simulink model "Gesamtsystem"  (R2018b)
settings: Solver=FixedStepDiscrete  StartTime=0.0  StopTime=1  RelTol=1e-3  EnableMultiTasking=on
libraries: commutil2 x12, c280xlib x8, c2833xlib x5, powerlib_extras x2, c2000lib x1
(part 1 of 2)
settings Model: ExtModeTrigDuration=8  Creator=User  LastModifiedBy=User
settings DataIOCC: LimitDataPoints=on  SaveFormat=Array  SaveOutput=off  SaveTime=off
settings OptimizationCC: DefaultUnderspecifiedDataType=single  ExpressionDepthLimit=2147483647  LifeSpan=1  MaxStackSize=512
settings DebuggingCC: UnderspecifiedInitializationDetection=Classic  MergeDetectMultiDrivingBlocksExec=none  SolverPrmCheckMsg=warning  StateNameClashWarn=warning  SFUnexpectedBacktrackingDiag=warning  SFNoUnconditionalDefaultTransitionDiag=warning  SFExecutionAtInitializationDiag=none
settings HardwareCC: ProdBitPerChar=16  ProdBitPerInt=16  ProdBitPerPointer=32  ProdBitPerSizeT=32  ProdBitPerPtrDiffT=32  ProdLargestAtomicInteger=Integer  ProdLargestAtomicFloat=None  ProdWordSize=16  ProdLongLongMode=on  ProdHWDeviceType=Texas Instruments->C2000  TargetBitPerChar=16  TargetBitPerInt=16  TargetLargestAtomicInteger=Integer  TargetIntDivRoundTo=Zero  TargetEndianess=LittleEndian  TargetWordSize=16  TargetHWDeviceType=Texas Instruments->C2000  ProdEqTarget=off
settings ModelReferenceCC: PropagateSignalLabelsOutOfModel=off
settings SFSimCC: SimCustomSourceCode="#include \"i2c_reset.c\""  SimCustomHeaderCode="#include \"i2c_reset.h\""  SimUseLocalCustomCode=off  MATLABDynamicMemAlloc=off
settings RTWCC: SystemTargetFile=ert.tlc  HardwareBoard=TI Delfino F2833x  TemplateMakefile=ert_default_tmf  RTWUseLocalCustomCode=off  RTWUseSimCustomCode=on  CustomSourceCode="#include \"i2c_reset.c\""  CustomHeaderCode="#include \"i2c_reset.h\""  Toolchain=Texas Instruments Code Composer Studio (C2000)
settings CodeAppCC: IgnoreCustomStorageClasses=off  CustomSymbolStrType=$N$R$M  StateflowObjectComments=on  InternalIdentifier=Classic
settings ERTTargetCC: CodeReplacementLibrary=TI C28x  MultiwordLength=2048  ParMdlRefBuildCompliant=off  CPPClassGenCompliant=off  ConvertIfToSwitch=off  SuppressUnreachableDefaultCases=off
settings ConfigComp: CovMetricSettings=dw  CovHtmlReporting=on  CovSaveCumulativeToWorkspaceVar=on  CovSaveSingleToWorkspaceVar=on  CovExternalEMLEnable=off  PSAutoStubLUT=on

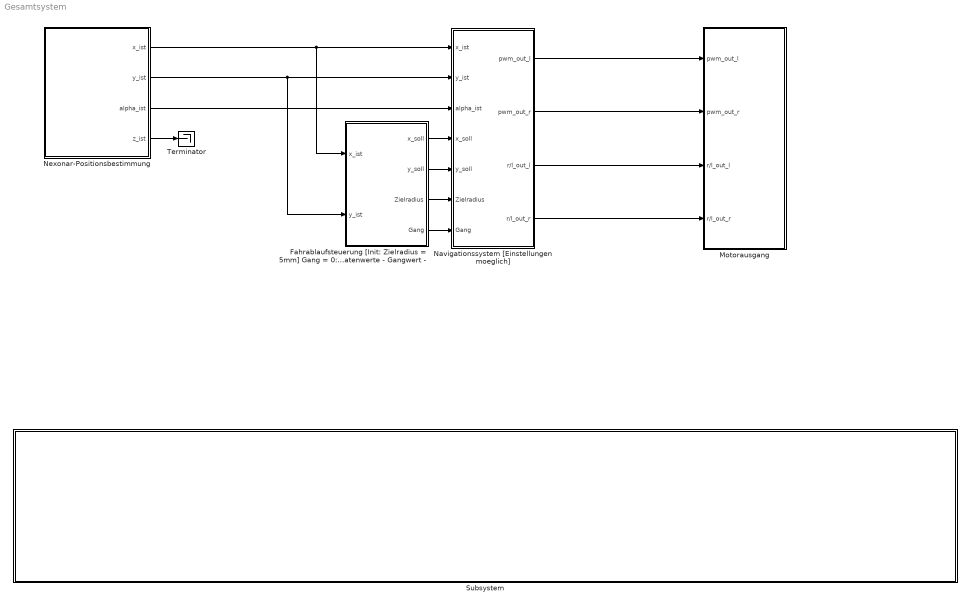
== system Gesamtsystem ==
  "Fahrablaufsteuerung [Init: Zielradius = 5mm] Gang = 0: vorwaerts Gang = 1: rueckwaerts Folgende Werte fuer den Ablauf sind einstellbar: - Zielkoordinatenwerte - Gangwert - " : Stateflow chart  TreatAsAtomicUnit=on
  Motorausgang : Subsystem
  Navigationssystem [Einstellungen moeglich] : Subsystem  TreatAsAtomicUnit=on
  Nexonar-Positionsbestimmung : Subsystem
  Subsystem : Subsystem
  Terminator : Terminator
  wires:
  "Fahrablaufsteuerung [Init: Zielradius = 5mm] Gang = 0: vorwaerts Gang = 1: rueckwaerts Folgende Werte fuer den Ablauf sind einstellbar: - Zielkoordinatenwerte - Gangwert - "/4(Gang) -> Navigationssystem [Einstellungen moeglich]/7(Gang)
  Nexonar-Positionsbestimmung/1(x_ist) -> "Fahrablaufsteuerung [Init: Zielradius = 5mm] Gang = 0: vorwaerts Gang = 1: rueckwaerts Folgende Werte fuer den Ablauf sind einstellbar: - Zielkoordinatenwerte - Gangwert - "/1(x_ist), Navigationssystem [Einstellungen moeglich]/1(x_ist)
  Nexonar-Positionsbestimmung/4(z_ist) -> Terminator/1
  Navigationssystem [Einstellungen moeglich]/4(r/l_out_r) -> Motorausgang/4(r/l_out_r)
  Navigationssystem [Einstellungen moeglich]/1(pwm_out_l) -> Motorausgang/1(pwm_out_l)
  Nexonar-Positionsbestimmung/2(y_ist) -> "Fahrablaufsteuerung [Init: Zielradius = 5mm] Gang = 0: vorwaerts Gang = 1: rueckwaerts Folgende Werte fuer den Ablauf sind einstellbar: - Zielkoordinatenwerte - Gangwert - "/2(y_ist), Navigationssystem [Einstellungen moeglich]/2(y_ist)
  "Fahrablaufsteuerung [Init: Zielradius = 5mm] Gang = 0: vorwaerts Gang = 1: rueckwaerts Folgende Werte fuer den Ablauf sind einstellbar: - Zielkoordinatenwerte - Gangwert - "/3(Zielradius) -> Navigationssystem [Einstellungen moeglich]/6(Zielradius)
  "Fahrablaufsteuerung [Init: Zielradius = 5mm] Gang = 0: vorwaerts Gang = 1: rueckwaerts Folgende Werte fuer den Ablauf sind einstellbar: - Zielkoordinatenwerte - Gangwert - "/1(x_soll) -> Navigationssystem [Einstellungen moeglich]/4(x_soll)
  Navigationssystem [Einstellungen moeglich]/2(pwm_out_r) -> Motorausgang/2(pwm_out_r)
  Nexonar-Positionsbestimmung/3(alpha_ist) -> Navigationssystem [Einstellungen moeglich]/3(alpha_ist)
  "Fahrablaufsteuerung [Init: Zielradius = 5mm] Gang = 0: vorwaerts Gang = 1: rueckwaerts Folgende Werte fuer den Ablauf sind einstellbar: - Zielkoordinatenwerte - Gangwert - "/2(y_soll) -> Navigationssystem [Einstellungen moeglich]/5(y_soll)
  Navigationssystem [Einstellungen moeglich]/3(r/l_out_l) -> Motorausgang/3(r/l_out_l)

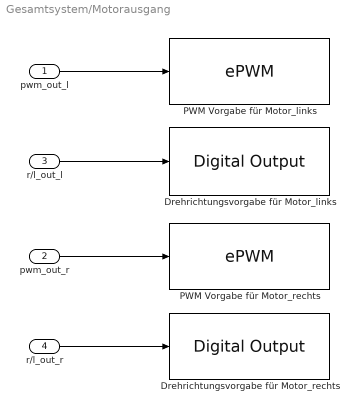
== system Gesamtsystem/Motorausgang ==
  pwm_out_l : Inport
  pwm_out_r : Inport  Port=2
  r/l_out_l : Inport  Port=3
  r/l_out_r : Inport  Port=4
  Drehrichtungsvorgabe für Motor_links : c2833xlib/Digital Output  GPIO_Number=GPIO16~GPIO23  GPIO_Bit0=off  GPIO_BIT0_Toggle=off  GPIO_Bit1=off  GPIO_BIT1_Toggle=off  GPIO_Bit2=off  GPIO_BIT2_Toggle=off  GPIO_Bit3=off  GPIO_BIT3_Toggle=off  GPIO_Bit4=off  GPIO_BIT4_Toggle=off  GPIO_Bit5=on  GPIO_BIT5_Toggle=off  GPIO_Bit6=off  GPIO_BIT6_Toggle=off  GPIO_Bit7=off  GPIO_BIT7_Toggle=off
      settings: SourceProductName=Embedded Coder Support Package for Texas Instruments C2000 Processors  SourceProductBaseCode=TIC2000
  Drehrichtungsvorgabe für Motor_rechts : c2833xlib/Digital Output  GPIO_Number=GPIO16~GPIO23  GPIO_Bit0=off  GPIO_BIT0_Toggle=off  GPIO_Bit1=off  GPIO_BIT1_Toggle=off  GPIO_Bit2=off  GPIO_BIT2_Toggle=off  GPIO_Bit3=off  GPIO_BIT3_Toggle=off  GPIO_Bit4=on  GPIO_BIT4_Toggle=off  GPIO_Bit5=off  GPIO_BIT5_Toggle=off  GPIO_Bit6=off  GPIO_BIT6_Toggle=off  GPIO_Bit7=off  GPIO_BIT7_Toggle=off
      settings: SourceProductName=Embedded Coder Support Package for Texas Instruments C2000 Processors  SourceProductBaseCode=TIC2000
  "PWM Vorgabe für Motor_links " : c280xlib/ePWM  checkMode=off  useModule=ePWM2  periodUnits=Clock cycles  timerSource=Specify via dialog  timerPeriod_clk=64000  timerPeriod_sec=0.0001  tbshadow=Counter equals to zero  countingMode=Up  phaseActiveEnable=Disable  phaseDirection=Count down after sync  phaseActive=0  synchronizationEnable=off  synchronizationOption=Disable  clockPrescale=1  HSclockPrescale=1  ePWMxAStatus=off  CMPAUnits=Clock cycles  CMPASource=Specify via dialog  CMPAValue_per=50  CMPAValue_clk=32000  enCMPAshadow=Counter equals to zero  ePWMxAactionLogic1=Do nothing  ePWMxAactionLogic2=Clear  ePWMxAactionLogic3=Set  ePWMxAactionLogic4=Do nothing  ePWMxAactionLogic5=Do nothing  ePWMxAactionLogic6=Do nothing  ePWMxALoadMode=Load on counter equals to zero (CTR=Zero)  ePWMxACSFenable=off  ePWMxACSFvalue=Forcing disable  ePWMxASFreload=Zero  enHRPWM=off  HRPWM_LoadMode=Counter equals to zero (CTR=ZERO)  HRPWM_CTLMode=Phase control mode  HRPWM_EDGMode=Both edge  enSFO=on  ePWMxBStatus=on  CMPBUnits=Percentages  CMPBSource=Input port  CMPBValue_per=0  CMPBValue_clk=32000  enCMPBshadow=Counter equals to zero  ePWMxBactionLogic1=Do nothing  ePWMxBactionLogic2=Set  ePWMxBactionLogic3=Do nothing  ePWMxBactionLogic4=Do nothing  ePWMxBactionLogic5=Clear  ePWMxBactionLogic6=Do nothing  ePWMxBLoadMode=Load on counter equals to zero (CTR=Zero)  ePWMxBCSFenable=off  ePWMxBCSFvalue=Forcing disable  ePWMxBSFreload=Zero  enableDBePWMxA=off  enableDBePWMxB=off  DBpolarity=Active high (AH)  DBedgeDelay=Positive  DBSource_ePWMxA=ePWMxA  DBSource_ePWMxB=ePWMxA  DBperiodSource=Specify via dialog  REDperiod=0  FEDperiod=0  adcstartModuleA=off  adcrequestEventA=First event  adcstartEventA=Counter equals to zero (CTR=Zero)  adcstartModuleB=off  adcrequestEventB=First event  adcstartEventB=Counter equals to zero (CTR=Zero)  intEn=off  intPrd=First event  intSel=Counter equals to zero (CTR=Zero)  chopperEnable=off  chopperFrequency=1  chopperFirstwidth=1  chopperDuty=12.5%  tripZonesource=Specify via dialog  tzselOSHT1=off  tzselOSHT2=off  tzselOSHT3=off  tzselOSHT4=off  tzselOSHT5=off  tzselOSHT6=off  tzselCBC1=off  tzselCBC2=off  tzselCBC3=off  tzselCBC4=off  tzselCBC5=off  tzselCBC6=off  enTzOstIntr=off  enTzCbcIntr=off  ePWMxAforced=No action  ePWMxBforced=No action  timerPeriod=-1  ePWMxAValue=0  ePWMxBValue=0  tripZoneoption=One-shot trip (OSHT)
      settings: SourceProductName=Embedded Coder Support Package for Texas Instruments C2000 Processors  SourceProductBaseCode=TIC2000
  PWM Vorgabe für Motor_rechts : c280xlib/ePWM  checkMode=off  useModule=ePWM1  periodUnits=Clock cycles  timerSource=Specify via dialog  timerPeriod_clk=64000  timerPeriod_sec=0.0001  tbshadow=Counter equals to zero  countingMode=Up  phaseActiveEnable=Disable  phaseDirection=Count down after sync  phaseActive=0  synchronizationEnable=off  synchronizationOption=Disable  clockPrescale=1  HSclockPrescale=1  ePWMxAStatus=off  CMPAUnits=Clock cycles  CMPASource=Specify via dialog  CMPAValue_per=50  CMPAValue_clk=32000  enCMPAshadow=Counter equals to zero  ePWMxAactionLogic1=Do nothing  ePWMxAactionLogic2=Clear  ePWMxAactionLogic3=Set  ePWMxAactionLogic4=Do nothing  ePWMxAactionLogic5=Do nothing  ePWMxAactionLogic6=Do nothing  ePWMxALoadMode=Load on counter equals to zero (CTR=Zero)  ePWMxACSFenable=off  ePWMxACSFvalue=Forcing disable  ePWMxASFreload=Zero  enHRPWM=off  HRPWM_LoadMode=Counter equals to zero (CTR=ZERO)  HRPWM_CTLMode=Phase control mode  HRPWM_EDGMode=Both edge  enSFO=on  ePWMxBStatus=on  CMPBUnits=Percentages  CMPBSource=Input port  CMPBValue_per=0  CMPBValue_clk=32000  enCMPBshadow=Counter equals to zero  ePWMxBactionLogic1=Do nothing  ePWMxBactionLogic2=Set  ePWMxBactionLogic3=Do nothing  ePWMxBactionLogic4=Do nothing  ePWMxBactionLogic5=Clear  ePWMxBactionLogic6=Do nothing  ePWMxBLoadMode=Load on counter equals to zero (CTR=Zero)  ePWMxBCSFenable=off  ePWMxBCSFvalue=Forcing disable  ePWMxBSFreload=Zero  enableDBePWMxA=off  enableDBePWMxB=off  DBpolarity=Active high (AH)  DBedgeDelay=Positive  DBSource_ePWMxA=ePWMxA  DBSource_ePWMxB=ePWMxA  DBperiodSource=Specify via dialog  REDperiod=0  FEDperiod=0  adcstartModuleA=off  adcrequestEventA=First event  adcstartEventA=Counter equals to zero (CTR=Zero)  adcstartModuleB=off  adcrequestEventB=First event  adcstartEventB=Counter equals to zero (CTR=Zero)  intEn=off  intPrd=First event  intSel=Counter equals to zero (CTR=Zero)  chopperEnable=off  chopperFrequency=1  chopperFirstwidth=1  chopperDuty=12.5%  tripZonesource=Specify via dialog  tzselOSHT1=off  tzselOSHT2=off  tzselOSHT3=off  tzselOSHT4=off  tzselOSHT5=off  tzselOSHT6=off  tzselCBC1=off  tzselCBC2=off  tzselCBC3=off  tzselCBC4=off  tzselCBC5=off  tzselCBC6=off  enTzOstIntr=off  enTzCbcIntr=off  ePWMxAforced=No action  ePWMxBforced=No action  timerPeriod=-1  ePWMxAValue=0  ePWMxBValue=0  tripZoneoption=One-shot trip (OSHT)
      settings: SourceProductName=Embedded Coder Support Package for Texas Instruments C2000 Processors  SourceProductBaseCode=TIC2000
  wires:
  pwm_out_l/1 -> "PWM Vorgabe für Motor_links "/1
  pwm_out_r/1 -> PWM Vorgabe für Motor_rechts/1
  r/l_out_l/1 -> Drehrichtungsvorgabe für Motor_links/1
  r/l_out_r/1 -> Drehrichtungsvorgabe für Motor_rechts/1

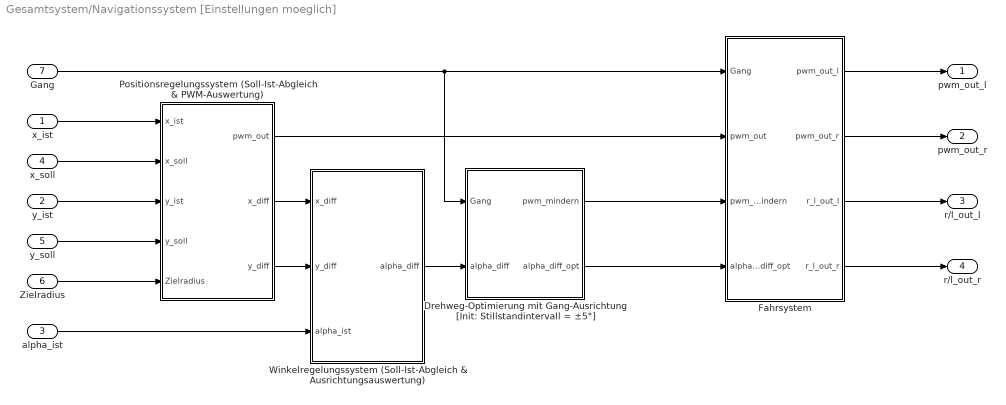
== system Gesamtsystem/Navigationssystem [Einstellungen moeglich] ==
  x_ist : Inport
  y_ist : Inport  Port=2
  alpha_ist : Inport  Port=3
  x_soll : Inport  Port=4
  y_soll : Inport  Port=5
  Zielradius : Inport  Port=6
  Gang : Inport  Port=7
  Drehweg-Optimierung mit Gang-Ausrichtung [Init: Stillstandintervall = ±5°] : Stateflow chart  TreatAsAtomicUnit=on
  Fahrsystem : Stateflow chart  TreatAsAtomicUnit=on
  Positionsregelungssystem (Soll-Ist-Abgleich & PWM-Auswertung) : Subsystem
  Winkelregelungssystem (Soll-Ist-Abgleich & Ausrichtungsauswertung) : Subsystem
  pwm_out_l : Outport
  pwm_out_r : Outport  Port=2
  r/l_out_l : Outport  Port=3
  r/l_out_r : Outport  Port=4
  wires:
  Positionsregelungssystem (Soll-Ist-Abgleich & PWM-Auswertung)/2(x_diff) -> Winkelregelungssystem (Soll-Ist-Abgleich & Ausrichtungsauswertung)/1(x_diff)
  y_soll/1 -> Positionsregelungssystem (Soll-Ist-Abgleich & PWM-Auswertung)/4(y_soll)
  y_ist/1 -> Positionsregelungssystem (Soll-Ist-Abgleich & PWM-Auswertung)/3(y_ist)
  Gang/1 -> Fahrsystem/1(Gang), Drehweg-Optimierung mit Gang-Ausrichtung [Init: Stillstandintervall = ±5°]/1(Gang)
  Positionsregelungssystem (Soll-Ist-Abgleich & PWM-Auswertung)/3(y_diff) -> Winkelregelungssystem (Soll-Ist-Abgleich & Ausrichtungsauswertung)/2(y_diff)
  x_ist/1 -> Positionsregelungssystem (Soll-Ist-Abgleich & PWM-Auswertung)/1(x_ist)
  x_soll/1 -> Positionsregelungssystem (Soll-Ist-Abgleich & PWM-Auswertung)/2(x_soll)
  alpha_ist/1 -> Winkelregelungssystem (Soll-Ist-Abgleich & Ausrichtungsauswertung)/3(alpha_ist)
  Fahrsystem/2(pwm_out_r) -> pwm_out_r/1
  Fahrsystem/4(r_l_out_r) -> r/l_out_r/1
  Fahrsystem/1(pwm_out_l) -> pwm_out_l/1
  Fahrsystem/3(r_l_out_l) -> r/l_out_l/1
  Winkelregelungssystem (Soll-Ist-Abgleich & Ausrichtungsauswertung)/1(alpha_diff) -> Drehweg-Optimierung mit Gang-Ausrichtung [Init: Stillstandintervall = ±5°]/2(alpha_diff)
  Drehweg-Optimierung mit Gang-Ausrichtung [Init: Stillstandintervall = ±5°]/2(alpha_diff_opt) -> Fahrsystem/4(alpha_diff_opt)
  Zielradius/1 -> Positionsregelungssystem (Soll-Ist-Abgleich & PWM-Auswertung)/5(Zielradius)
  Drehweg-Optimierung mit Gang-Ausrichtung [Init: Stillstandintervall = ±5°]/1(pwm_mindern) -> Fahrsystem/3(pwm_mindern)
  Positionsregelungssystem (Soll-Ist-Abgleich & PWM-Auswertung)/1(pwm_out) -> Fahrsystem/2(pwm_out)

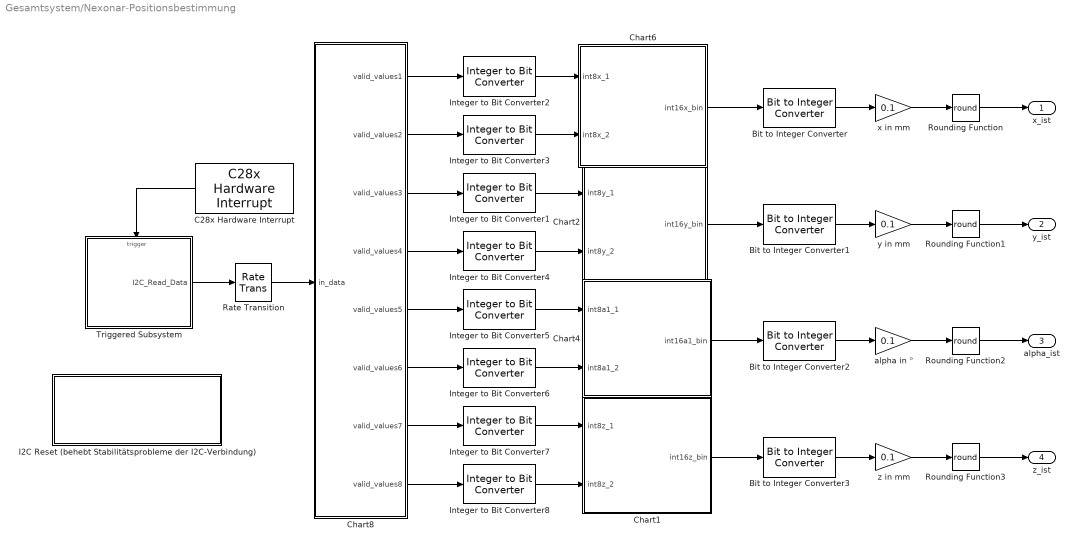
== system Gesamtsystem/Nexonar-Positionsbestimmung ==
  Bit to Integer Converter{,1..3} (4 alike) : commutil2/Bit to Integer Converter  nbits=16  bitOrder=MSB first  signedOutputValues=Signed  outDtype=Inherit via internal rule  outDtypeSigned=Inherit via internal rule
      settings: SourceProductName=Communications Toolbox
  C28x Hardware Interrupt : c2000lib/Scheduling/C28x Hardware Interrupt  irqnumbers=8  pienumbers=2  irqpriorities=30  irqpreempts=0  showinput=off  dspchiptype=C280X
      settings: SourceProductName=Embedded Coder Support Package for Texas Instruments C2000 Processors  SourceProductBaseCode=TIC2000
  Chart1 : Stateflow chart  TreatAsAtomicUnit=on
  Chart2 : Stateflow chart  TreatAsAtomicUnit=on
  Chart4 : Stateflow chart  TreatAsAtomicUnit=on
  Chart6 : Stateflow chart  TreatAsAtomicUnit=on
  Chart8 : Stateflow chart  TreatAsAtomicUnit=on
  I2C Reset (behebt Stabilitätsprobleme der I2C-Verbindung) : Subsystem
  Integer to Bit Converter{1..8} (8 alike) : commutil2/Integer to Bit Converter  nbits=8  signedInputValues=Unsigned  bitOrder=MSB first  outDtype=uint8
      settings: SourceProductName=Communications Toolbox
  Rate Transition : RateTransition  Deterministic=off  OutPortSampleTime=0.01
  Rounding Function{,1..3} (4 alike) : Rounding  Operator=round
  Triggered Subsystem : Subsystem  TreatAsAtomicUnit=on
  alpha in ° : Gain  Gain=0.1  OutDataTypeStr=double
  x in mm : Gain  Gain=0.1  OutDataTypeStr=double
  y in mm : Gain  Gain=0.1  OutDataTypeStr=double
  z in mm : Gain  Gain=0.1  OutDataTypeStr=double
  x_ist : Outport
  y_ist : Outport  Port=2
  alpha_ist : Outport  Port=3
  z_ist : Outport  Port=4
  wires:
  Integer to Bit Converter7/1 -> Chart1/1(int8z_1)
  Integer to Bit Converter8/1 -> Chart1/2(int8z_2)
  Chart8/7(valid_values7) -> Integer to Bit Converter7/1
  Chart8/8(valid_values8) -> Integer to Bit Converter8/1
  Triggered Subsystem/1(I2C_Read_Data) -> Rate Transition/1
  Chart1/1(int16z_bin) -> Bit to Integer Converter3/1
  Chart4/1(int16a1_bin) -> Bit to Integer Converter2/1
  Chart8/6(valid_values6) -> Integer to Bit Converter6/1
  Integer to Bit Converter6/1 -> Chart4/2(int8a1_2)
  Integer to Bit Converter5/1 -> Chart4/1(int8a1_1)
  Integer to Bit Converter4/1 -> Chart2/2(int8y_2)
  Integer to Bit Converter2/1 -> Chart6/1(int8x_1)
  Integer to Bit Converter1/1 -> Chart2/1(int8y_1)
  Chart6/1(int16x_bin) -> Bit to Integer Converter/1
  Integer to Bit Converter3/1 -> Chart6/2(int8x_2)
  Chart8/3(valid_values3) -> Integer to Bit Converter1/1
  Chart8/1(valid_values1) -> Integer to Bit Converter2/1
  Chart2/1(int16y_bin) -> Bit to Integer Converter1/1
  Chart8/4(valid_values4) -> Integer to Bit Converter4/1
  Chart8/2(valid_values2) -> Integer to Bit Converter3/1
  Chart8/5(valid_values5) -> Integer to Bit Converter5/1
  C28x Hardware Interrupt/1 -> Triggered Subsystem/Trigger
  Rate Transition/1 -> Chart8/1(in_data)
  x in mm/1 -> Rounding Function/1
  Bit to Integer Converter/1 -> x in mm/1
  Bit to Integer Converter1/1 -> y in mm/1
  y in mm/1 -> Rounding Function1/1
  Bit to Integer Converter3/1 -> z in mm/1
  z in mm/1 -> Rounding Function3/1
  Bit to Integer Converter2/1 -> alpha in °/1
  alpha in °/1 -> Rounding Function2/1
  Rounding Function/1 -> x_ist/1
  Rounding Function2/1 -> alpha_ist/1
  Rounding Function1/1 -> y_ist/1
  Rounding Function3/1 -> z_ist/1

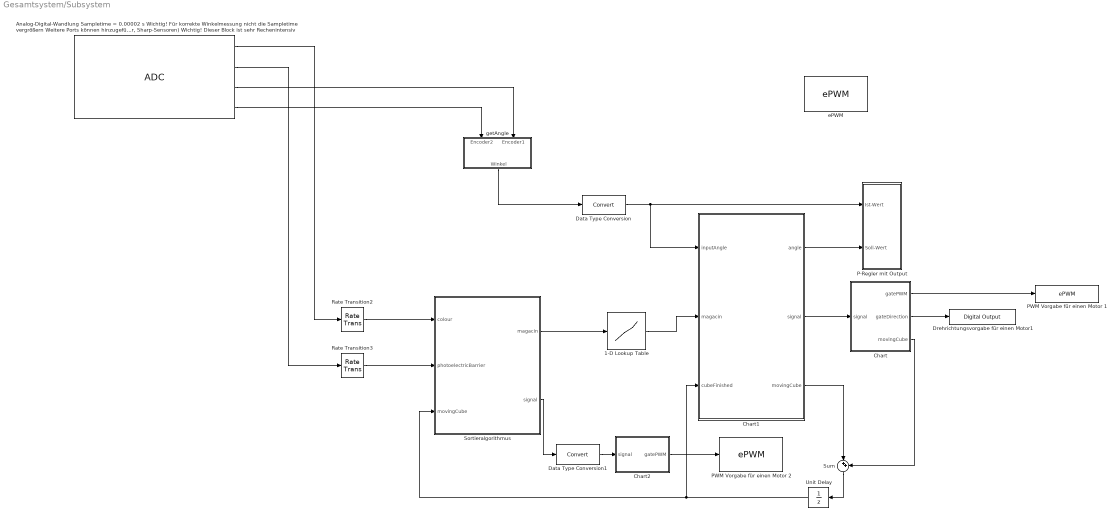
== system Gesamtsystem/Subsystem ==
  1-D Lookup Table : Lookup_n-D  NumberOfTableDimensions=1  BreakpointsForDimension1=[-1,0,1,2,3,4,5,6]  Table=[-1,-440,-295,-170,-40,85,220,430]  InternalRulePriority=Speed  RndMeth=Simplest  InputSameDT=on
  "Analog-Digital-Wandlung Sampletime = 0.00002 s Wichtig! Für korrekte Winkelmessung nicht die Sampletime vergrößern Weitere Ports können hinzugefügt werden (Farbsensor, Sharp-Sensoren) Wichtig! Dieser Block ist sehr Rechenintensiv" : c280xlib/ADC  useModule=A  useMode=Sequential  sourceSOC=Software  sourceSOC1=Software  sourceSOC2=ePWMxB  xint2_ADCSOC=31  Ts=0.00002  dType=double  postInterrupt=off  numConversionsSingle=4  numConversionsDouble=1  conv0=ADCINA0  conv1=ADCINA1  conv2=ADCINA2  conv3=ADCINA3  conv4=ADCINA4  conv5=ADCINA5  conv6=ADCINA6  conv7=ADCINA7  conv8=ADCINB0  conv9=ADCINB1  conv10=ADCINB2  conv11=ADCINB3  conv12=ADCINB4  conv13=ADCINB5  conv14=ADCINB6  conv15=ADCINB7  convAB0=ADCINA0 and ADCINB0  convAB1=ADCINA1 and ADCINB1  convAB2=ADCINA2 and ADCINB2  convAB3=ADCINA3 and ADCINB3  convAB4=ADCINA4 and ADCINB4  convAB5=ADCINA5 and ADCINB5  convAB6=ADCINA6 and ADCINB6  convAB7=ADCINA7 and ADCINB7  convA0=ADCINA5  convA1=ADCINA4  convA2=ADCINA0  convA3=ADCINA1  convA4=ADCINA5  convA5=ADCINA5  convA6=ADCINA6  convA7=ADCINA7  convB0=ADCINB0  convB1=ADCINB1  convB2=ADCINB2  convB3=ADCINB3  convB4=ADCINB4  convB5=ADCINB5  convB6=ADCINB6  convB7=ADCINB7  c28xmultiPort=on  endma=off  chdma=1
      settings: SourceProductName=Embedded Coder Support Package for Texas Instruments C2000 Processors  SourceProductBaseCode=TIC2000
  Chart : Stateflow chart  TreatAsAtomicUnit=on
  Chart1 : Stateflow chart  TreatAsAtomicUnit=on
  Chart2 : Stateflow chart  TreatAsAtomicUnit=on
  Data Type Conversion : DataTypeConversion
  Data Type Conversion1 : DataTypeConversion
  Drehrichtungsvorgabe für einen Motor1 : c2833xlib/Digital Output  GPIO_Number=GPIO16~GPIO23  GPIO_Bit0=on  GPIO_BIT0_Toggle=off  GPIO_Bit1=off  GPIO_BIT1_Toggle=off  GPIO_Bit2=off  GPIO_BIT2_Toggle=off  GPIO_Bit3=off  GPIO_BIT3_Toggle=off  GPIO_Bit4=off  GPIO_BIT4_Toggle=off  GPIO_Bit5=off  GPIO_BIT5_Toggle=off  GPIO_Bit6=off  GPIO_BIT6_Toggle=off  GPIO_Bit7=off  GPIO_BIT7_Toggle=off
      settings: SourceProductName=Embedded Coder Support Package for Texas Instruments C2000 Processors  SourceProductBaseCode=TIC2000
  P-Regler mit Output : Subsystem
  PWM Vorgabe für einen Motor 1 : c280xlib/ePWM  checkMode=off  useModule=ePWM6  periodUnits=Clock cycles  timerSource=Specify via dialog  timerPeriod_clk=64000  timerPeriod_sec=0.0001  tbshadow=Counter equals to zero  countingMode=Up  phaseActiveEnable=Disable  phaseDirection=Count down after sync  phaseActive=0  synchronizationEnable=off  synchronizationOption=Disable  clockPrescale=1  HSclockPrescale=1  ePWMxAStatus=off  CMPAUnits=Clock cycles  CMPASource=Specify via dialog  CMPAValue_per=50  CMPAValue_clk=32000  enCMPAshadow=Counter equals to zero  ePWMxAactionLogic1=Do nothing  ePWMxAactionLogic2=Clear  ePWMxAactionLogic3=Set  ePWMxAactionLogic4=Do nothing  ePWMxAactionLogic5=Do nothing  ePWMxAactionLogic6=Do nothing  ePWMxALoadMode=Load on counter equals to zero (CTR=Zero)  ePWMxACSFenable=off  ePWMxACSFvalue=Forcing disable  ePWMxASFreload=Zero  enHRPWM=off  HRPWM_LoadMode=Counter equals to zero (CTR=ZERO)  HRPWM_CTLMode=Phase control mode  HRPWM_EDGMode=Both edge  enSFO=on  ePWMxBStatus=on  CMPBUnits=Percentages  CMPBSource=Input port  CMPBValue_per=0  CMPBValue_clk=32000  enCMPBshadow=Counter equals to zero  ePWMxBactionLogic1=Do nothing  ePWMxBactionLogic2=Set  ePWMxBactionLogic3=Do nothing  ePWMxBactionLogic4=Do nothing  ePWMxBactionLogic5=Clear  ePWMxBactionLogic6=Do nothing  ePWMxBLoadMode=Load on counter equals to zero (CTR=Zero)  ePWMxBCSFenable=off  ePWMxBCSFvalue=Forcing disable  ePWMxBSFreload=Zero  enableDBePWMxA=off  enableDBePWMxB=off  DBpolarity=Active high (AH)  DBedgeDelay=Positive  DBSource_ePWMxA=ePWMxA  DBSource_ePWMxB=ePWMxA  DBperiodSource=Specify via dialog  REDperiod=0  FEDperiod=0  adcstartModuleA=off  adcrequestEventA=First event  adcstartEventA=Counter equals to zero (CTR=Zero)  adcstartModuleB=off  adcrequestEventB=First event  adcstartEventB=Counter equals to zero (CTR=Zero)  intEn=off  intPrd=First event  intSel=Counter equals to zero (CTR=Zero)  chopperEnable=off  chopperFrequency=1  chopperFirstwidth=1  chopperDuty=12.5%  tripZonesource=Specify via dialog  tzselOSHT1=off  tzselOSHT2=off  tzselOSHT3=off  tzselOSHT4=off  tzselOSHT5=off  tzselOSHT6=off  tzselCBC1=off  tzselCBC2=off  tzselCBC3=off  tzselCBC4=off  tzselCBC5=off  tzselCBC6=off  enTzOstIntr=off  enTzCbcIntr=off  ePWMxAforced=No action  ePWMxBforced=No action  timerPeriod=-1  ePWMxAValue=0  ePWMxBValue=0  tripZoneoption=One-shot trip (OSHT)
      settings: SourceProductName=Embedded Coder Support Package for Texas Instruments C2000 Processors  SourceProductBaseCode=TIC2000
  PWM Vorgabe für einen Motor 2 : c280xlib/ePWM  checkMode=off  useModule=ePWM3  periodUnits=Clock cycles  timerSource=Specify via dialog  timerPeriod_clk=64000  timerPeriod_sec=0.0001  tbshadow=Counter equals to zero  countingMode=Up  phaseActiveEnable=Disable  phaseDirection=Count down after sync  phaseActive=0  synchronizationEnable=off  synchronizationOption=Disable  clockPrescale=1  HSclockPrescale=1  ePWMxAStatus=off  CMPAUnits=Clock cycles  CMPASource=Specify via dialog  CMPAValue_per=50  CMPAValue_clk=32000  enCMPAshadow=Counter equals to zero  ePWMxAactionLogic1=Do nothing  ePWMxAactionLogic2=Clear  ePWMxAactionLogic3=Set  ePWMxAactionLogic4=Do nothing  ePWMxAactionLogic5=Do nothing  ePWMxAactionLogic6=Do nothing  ePWMxALoadMode=Load on counter equals to zero (CTR=Zero)  ePWMxACSFenable=off  ePWMxACSFvalue=Forcing disable  ePWMxASFreload=Zero  enHRPWM=off  HRPWM_LoadMode=Counter equals to zero (CTR=ZERO)  HRPWM_CTLMode=Phase control mode  HRPWM_EDGMode=Both edge  enSFO=on  ePWMxBStatus=on  CMPBUnits=Percentages  CMPBSource=Input port  CMPBValue_per=0  CMPBValue_clk=32000  enCMPBshadow=Counter equals to zero  ePWMxBactionLogic1=Do nothing  ePWMxBactionLogic2=Set  ePWMxBactionLogic3=Do nothing  ePWMxBactionLogic4=Do nothing  ePWMxBactionLogic5=Clear  ePWMxBactionLogic6=Do nothing  ePWMxBLoadMode=Load on counter equals to zero (CTR=Zero)  ePWMxBCSFenable=off  ePWMxBCSFvalue=Forcing disable  ePWMxBSFreload=Zero  enableDBePWMxA=off  enableDBePWMxB=off  DBpolarity=Active high (AH)  DBedgeDelay=Positive  DBSource_ePWMxA=ePWMxA  DBSource_ePWMxB=ePWMxA  DBperiodSource=Specify via dialog  REDperiod=0  FEDperiod=0  adcstartModuleA=off  adcrequestEventA=First event  adcstartEventA=Counter equals to zero (CTR=Zero)  adcstartModuleB=off  adcrequestEventB=First event  adcstartEventB=Counter equals to zero (CTR=Zero)  intEn=off  intPrd=First event  intSel=Counter equals to zero (CTR=Zero)  chopperEnable=off  chopperFrequency=1  chopperFirstwidth=1  chopperDuty=12.5%  tripZonesource=Specify via dialog  tzselOSHT1=off  tzselOSHT2=off  tzselOSHT3=off  tzselOSHT4=off  tzselOSHT5=off  tzselOSHT6=off  tzselCBC1=off  tzselCBC2=off  tzselCBC3=off  tzselCBC4=off  tzselCBC5=off  tzselCBC6=off  enTzOstIntr=off  enTzCbcIntr=off  ePWMxAforced=No action  ePWMxBforced=No action  timerPeriod=-1  ePWMxAValue=0  ePWMxBValue=0  tripZoneoption=One-shot trip (OSHT)
      settings: SourceProductName=Embedded Coder Support Package for Texas Instruments C2000 Processors  SourceProductBaseCode=TIC2000
  Rate Transition2 : RateTransition  OutPortSampleTime=0.01
  Rate Transition3 : RateTransition  OutPortSampleTime=0.01
  Sortieralgorithmus : Stateflow chart  TreatAsAtomicUnit=on
  Sum : Sum  Inputs=|++
  Unit Delay : UnitDelay  SampleTime=-1
  ePWM : c280xlib/ePWM  checkMode=off  useModule=ePWM5  periodUnits=Clock cycles  timerSource=Specify via dialog  timerPeriod_clk=64000  timerPeriod_sec=0.0001  tbshadow=Counter equals to zero  countingMode=Up  phaseActiveEnable=Disable  phaseDirection=Count down after sync  phaseActive=0  synchronizationEnable=off  synchronizationOption=Disable  clockPrescale=1  HSclockPrescale=1  ePWMxAStatus=off  CMPAUnits=Percentages  CMPASource=Specify via dialog  CMPAValue_per=30  CMPAValue_clk=32000  enCMPAshadow=Counter equals to zero  ePWMxAactionLogic1=Do nothing  ePWMxAactionLogic2=Clear  ePWMxAactionLogic3=Set  ePWMxAactionLogic4=Do nothing  ePWMxAactionLogic5=Do nothing  ePWMxAactionLogic6=Do nothing  ePWMxALoadMode=Load on counter equals to zero (CTR=Zero)  ePWMxACSFenable=off  ePWMxACSFvalue=Forcing disable  ePWMxASFreload=Zero  enHRPWM=off  HRPWM_LoadMode=Counter equals to zero (CTR=ZERO)  HRPWM_CTLMode=Phase control mode  HRPWM_EDGMode=Both edge  enSFO=on  ePWMxBStatus=on  CMPBUnits=Percentages  CMPBSource=Specify via dialog  CMPBValue_per=80  CMPBValue_clk=32000  enCMPBshadow=Counter equals to zero  ePWMxBactionLogic1=Do nothing  ePWMxBactionLogic2=Set  ePWMxBactionLogic3=Do nothing  ePWMxBactionLogic4=Do nothing  ePWMxBactionLogic5=Clear  ePWMxBactionLogic6=Do nothing  ePWMxBLoadMode=Load on counter equals to zero (CTR=Zero)  ePWMxBCSFenable=off  ePWMxBCSFvalue=Forcing disable  ePWMxBSFreload=Zero  enableDBePWMxA=off  enableDBePWMxB=off  DBpolarity=Active high (AH)  DBedgeDelay=Positive  DBSource_ePWMxA=ePWMxA  DBSource_ePWMxB=ePWMxA  DBperiodSource=Specify via dialog  REDperiod=0  FEDperiod=0  adcstartModuleA=off  adcrequestEventA=First event  adcstartEventA=Counter equals to zero (CTR=Zero)  adcstartModuleB=off  adcrequestEventB=First event  adcstartEventB=Counter equals to zero (CTR=Zero)  intEn=off  intPrd=First event  intSel=Counter equals to zero (CTR=Zero)  chopperEnable=off  chopperFrequency=1  chopperFirstwidth=1  chopperDuty=12.5%  tripZonesource=Specify via dialog  tzselOSHT1=off  tzselOSHT2=off  tzselOSHT3=off  tzselOSHT4=off  tzselOSHT5=off  tzselOSHT6=off  tzselCBC1=off  tzselCBC2=off  tzselCBC3=off  tzselCBC4=off  tzselCBC5=off  tzselCBC6=off  enTzOstIntr=off  enTzCbcIntr=off  ePWMxAforced=No action  ePWMxBforced=No action  timerPeriod=-1  ePWMxAValue=0  ePWMxBValue=0  tripZoneoption=One-shot trip (OSHT)
      settings: SourceProductName=Embedded Coder Support Package for Texas Instruments C2000 Processors  SourceProductBaseCode=TIC2000
  getAngle : Subsystem
  wires:
  Chart2/1(gatePWM) -> PWM Vorgabe für einen Motor 2/1
  "Analog-Digital-Wandlung Sampletime = 0.00002 s Wichtig! Für korrekte Winkelmessung nicht die Sampletime vergrößern Weitere Ports können hinzugefügt werden (Farbsensor, Sharp-Sensoren) Wichtig! Dieser Block ist sehr Rechenintensiv"/4 -> getAngle/1(Encoder2)
  "Analog-Digital-Wandlung Sampletime = 0.00002 s Wichtig! Für korrekte Winkelmessung nicht die Sampletime vergrößern Weitere Ports können hinzugefügt werden (Farbsensor, Sharp-Sensoren) Wichtig! Dieser Block ist sehr Rechenintensiv"/1 -> Rate Transition2/1
  "Analog-Digital-Wandlung Sampletime = 0.00002 s Wichtig! Für korrekte Winkelmessung nicht die Sampletime vergrößern Weitere Ports können hinzugefügt werden (Farbsensor, Sharp-Sensoren) Wichtig! Dieser Block ist sehr Rechenintensiv"/3 -> getAngle/2(Encoder1)
  Chart/1(gatePWM) -> PWM Vorgabe für einen Motor 1/1
  Sortieralgorithmus/1(magacin) -> 1-D Lookup Table/1
  Chart1/3(movingCube) -> Sum/1
  Chart1/2(signal) -> Chart/1(signal)
  Chart1/1(angle) -> P-Regler mit Output/2(Soll-Wert)
  Rate Transition3/1 -> Sortieralgorithmus/2(photoelectricBarrier)
  1-D Lookup Table/1 -> Chart1/2(magacin)
  Rate Transition2/1 -> Sortieralgorithmus/1(colour)
  Data Type Conversion1/1 -> Chart2/1(signal)
  Sortieralgorithmus/2(signal) -> Data Type Conversion1/1
  Chart/2(gateDirection) -> Drehrichtungsvorgabe für einen Motor1/1
  Chart/3(movingCube) -> Sum/2
  Data Type Conversion/1 -> Chart1/1(inputAngle), P-Regler mit Output/1(Ist-Wert)
  getAngle/1(Winkel) -> Data Type Conversion/1
  Unit Delay/1 -> Chart1/3(cubeFinished), Sortieralgorithmus/3(movingCube)
  "Analog-Digital-Wandlung Sampletime = 0.00002 s Wichtig! Für korrekte Winkelmessung nicht die Sampletime vergrößern Weitere Ports können hinzugefügt werden (Farbsensor, Sharp-Sensoren) Wichtig! Dieser Block ist sehr Rechenintensiv"/2 -> Rate Transition3/1
  Sum/1 -> Unit Delay/1

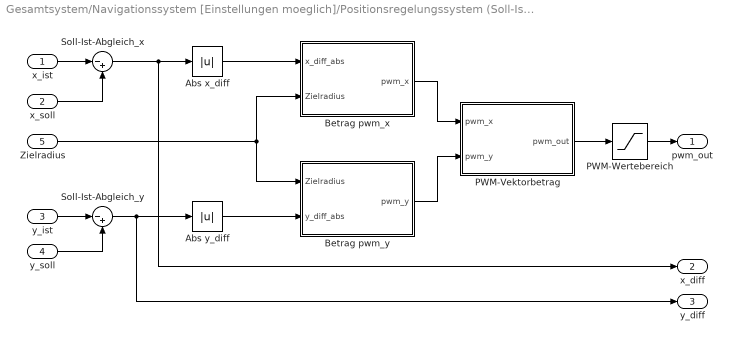
== system Gesamtsystem/Navigationssystem [Einstellungen moeglich]/Positionsregelungssystem (Soll-Ist-Abgleich & PWM-Auswertung) ==
  x_ist : Inport
  x_soll : Inport  Port=2
  y_ist : Inport  Port=3
  y_soll : Inport  Port=4
  Zielradius : Inport  Port=5
  Abs x_diff : Abs  SampleTime=0.01
  Abs y_diff : Abs  SampleTime=0.01
  Betrag pwm_x : MATLAB Function  TreatAsAtomicUnit=on  SystemSampleTime=0.01
  Betrag pwm_y : MATLAB Function  TreatAsAtomicUnit=on  SystemSampleTime=0.01
  PWM-Vektorbetrag : MATLAB Function  TreatAsAtomicUnit=on
  PWM-Wertebereich : Saturate  UpperLimit=100  LowerLimit=0
  Soll-Ist-Abgleich_x : Sum  Inputs=|-+  SampleTime=0.01
  Soll-Ist-Abgleich_y : Sum  Inputs=|-+  AccumDataTypeStr=double  SampleTime=0.01
  pwm_out : Outport
  x_diff : Outport  Port=2
  y_diff : Outport  Port=3
  wires:
  Soll-Ist-Abgleich_x/1 -> x_diff/1, Abs x_diff/1
  Abs x_diff/1 -> Betrag pwm_x/1(x_diff_abs)
  x_soll/1 -> Soll-Ist-Abgleich_x/2
  x_ist/1 -> Soll-Ist-Abgleich_x/1
  y_ist/1 -> Soll-Ist-Abgleich_y/1
  y_soll/1 -> Soll-Ist-Abgleich_y/2
  Soll-Ist-Abgleich_y/1 -> Abs y_diff/1, y_diff/1
  Abs y_diff/1 -> Betrag pwm_y/2(y_diff_abs)
  PWM-Wertebereich/1 -> pwm_out/1
  PWM-Vektorbetrag/1(pwm_out) -> PWM-Wertebereich/1
  Betrag pwm_x/1(pwm_x) -> PWM-Vektorbetrag/1(pwm_x)
  Betrag pwm_y/1(pwm_y) -> PWM-Vektorbetrag/2(pwm_y)
  Zielradius/1 -> Betrag pwm_y/1(Zielradius), Betrag pwm_x/2(Zielradius)

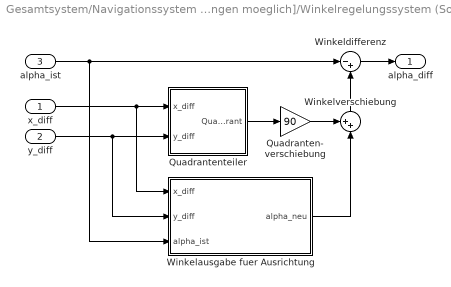
== system Gesamtsystem/Navigationssystem [Einstellungen moeglich]/Winkelregelungssystem (Soll-Ist-Abgleich & Ausrichtungsauswertung) ==
  x_diff : Inport
  y_diff : Inport  Port=2
  alpha_ist : Inport  Port=3
  Quadranten- verschiebung : Gain  Gain=90
  Quadrantenteiler : Stateflow chart  TreatAsAtomicUnit=on
  Winkelausgabe fuer Ausrichtung : Stateflow chart  TreatAsAtomicUnit=on
  Winkeldifferenz : Sum  Inputs=|-+
  Winkelverschiebung : Sum  Inputs=++|
  alpha_diff : Outport
  wires:
  alpha_ist/1 -> Winkelausgabe fuer Ausrichtung/3(alpha_ist), Winkeldifferenz/1
  y_diff/1 -> Winkelausgabe fuer Ausrichtung/2(y_diff), Quadrantenteiler/2(y_diff)
  Winkelausgabe fuer Ausrichtung/1(alpha_neu) -> Winkelverschiebung/2
  Winkelverschiebung/1 -> Winkeldifferenz/2
  x_diff/1 -> Winkelausgabe fuer Ausrichtung/1(x_diff), Quadrantenteiler/1(x_diff)
  Quadrantenteiler/1(Quadrant) -> Quadranten- verschiebung/1
  Winkeldifferenz/1 -> alpha_diff/1
  Quadranten- verschiebung/1 -> Winkelverschiebung/1

== system Gesamtsystem/Nexonar-Positionsbestimmung/I2C Reset (behebt Stabilitätsprobleme der I2C-Verbindung) ==
  I2C Reinitialisierung : Subsystem  TreatAsAtomicUnit=on
  I2C Reset : Subsystem  TreatAsAtomicUnit=on
  Pulse Generator : DiscretePulseGenerator  Period=250  SampleTime=0.01
  wires:
  Pulse Generator/1 -> I2C Reinitialisierung/Trigger, I2C Reset/Trigger

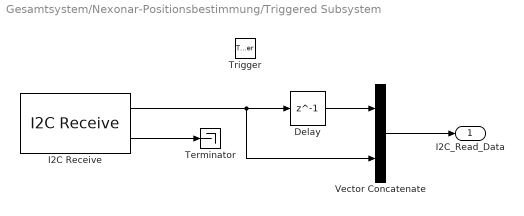
== system Gesamtsystem/Nexonar-Positionsbestimmung/Triggered Subsystem ==
  Trigger : TriggerPort  TriggerType=function-call  VariantControl=(inherit)
  Delay : Delay  DelayLength=1  InitialCondition=0
  I2C Receive : c280xlib/I2C Receive  selectModule=I2C_A  addrFormat=7-Bit addressing  saSource=Specify via dialog  SAR=80  bitCount=8  dataLength=10  initValue=0  NACK=on  STP=off  STR=on  sampleTime=-1  dataType=uint8
      settings: SourceProductName=Embedded Coder Support Package for Texas Instruments C2000 Processors  SourceProductBaseCode=TIC2000
  Terminator : Terminator
  Vector Concatenate : Concatenate
  I2C_Read_Data : Outport
  wires:
  I2C Receive/2 -> Terminator/1
  I2C Receive/1 -> Vector Concatenate/2, Delay/1
  Delay/1 -> Vector Concatenate/1
  Vector Concatenate/1 -> I2C_Read_Data/1

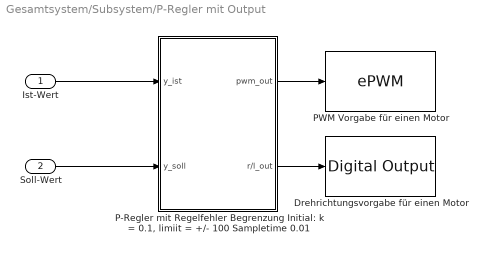
== system Gesamtsystem/Subsystem/P-Regler mit Output ==
  Ist-Wert : Inport
  Soll-Wert : Inport  Port=2
  Drehrichtungsvorgabe für einen Motor : c2833xlib/Digital Output  GPIO_Number=GPIO16~GPIO23  GPIO_Bit0=off  GPIO_BIT0_Toggle=off  GPIO_Bit1=off  GPIO_BIT1_Toggle=off  GPIO_Bit2=off  GPIO_BIT2_Toggle=off  GPIO_Bit3=on  GPIO_BIT3_Toggle=off  GPIO_Bit4=off  GPIO_BIT4_Toggle=off  GPIO_Bit5=off  GPIO_BIT5_Toggle=off  GPIO_Bit6=off  GPIO_BIT6_Toggle=off  GPIO_Bit7=off  GPIO_BIT7_Toggle=off
      settings: SourceProductName=Embedded Coder Support Package for Texas Instruments C2000 Processors  SourceProductBaseCode=TIC2000
  "P-Regler mit Regelfehler Begrenzung Initial: k = 0.1, limiit = +/- 100 Sampletime 0.01" : Subsystem
  "PWM Vorgabe für einen Motor " : c280xlib/ePWM  checkMode=off  useModule=ePWM4  periodUnits=Clock cycles  timerSource=Specify via dialog  timerPeriod_clk=64000  timerPeriod_sec=0.0001  tbshadow=Counter equals to zero  countingMode=Up  phaseActiveEnable=Disable  phaseDirection=Count down after sync  phaseActive=0  synchronizationEnable=off  synchronizationOption=Disable  clockPrescale=1  HSclockPrescale=1  ePWMxAStatus=off  CMPAUnits=Clock cycles  CMPASource=Specify via dialog  CMPAValue_per=50  CMPAValue_clk=32000  enCMPAshadow=Counter equals to zero  ePWMxAactionLogic1=Do nothing  ePWMxAactionLogic2=Clear  ePWMxAactionLogic3=Set  ePWMxAactionLogic4=Do nothing  ePWMxAactionLogic5=Do nothing  ePWMxAactionLogic6=Do nothing  ePWMxALoadMode=Load on counter equals to zero (CTR=Zero)  ePWMxACSFenable=off  ePWMxACSFvalue=Forcing disable  ePWMxASFreload=Zero  enHRPWM=off  HRPWM_LoadMode=Counter equals to zero (CTR=ZERO)  HRPWM_CTLMode=Phase control mode  HRPWM_EDGMode=Both edge  enSFO=on  ePWMxBStatus=on  CMPBUnits=Percentages  CMPBSource=Input port  CMPBValue_per=0  CMPBValue_clk=32000  enCMPBshadow=Counter equals to zero  ePWMxBactionLogic1=Do nothing  ePWMxBactionLogic2=Set  ePWMxBactionLogic3=Do nothing  ePWMxBactionLogic4=Do nothing  ePWMxBactionLogic5=Clear  ePWMxBactionLogic6=Do nothing  ePWMxBLoadMode=Load on counter equals to zero (CTR=Zero)  ePWMxBCSFenable=off  ePWMxBCSFvalue=Forcing disable  ePWMxBSFreload=Zero  enableDBePWMxA=off  enableDBePWMxB=off  DBpolarity=Active high (AH)  DBedgeDelay=Positive  DBSource_ePWMxA=ePWMxA  DBSource_ePWMxB=ePWMxA  DBperiodSource=Specify via dialog  REDperiod=0  FEDperiod=0  adcstartModuleA=off  adcrequestEventA=First event  adcstartEventA=Counter equals to zero (CTR=Zero)  adcstartModuleB=off  adcrequestEventB=First event  adcstartEventB=Counter equals to zero (CTR=Zero)  intEn=off  intPrd=First event  intSel=Counter equals to zero (CTR=Zero)  chopperEnable=off  chopperFrequency=1  chopperFirstwidth=1  chopperDuty=12.5%  tripZonesource=Specify via dialog  tzselOSHT1=off  tzselOSHT2=off  tzselOSHT3=off  tzselOSHT4=off  tzselOSHT5=off  tzselOSHT6=off  tzselCBC1=off  tzselCBC2=off  tzselCBC3=off  tzselCBC4=off  tzselCBC5=off  tzselCBC6=off  enTzOstIntr=off  enTzCbcIntr=off  ePWMxAforced=No action  ePWMxBforced=No action  timerPeriod=-1  ePWMxAValue=0  ePWMxBValue=0  tripZoneoption=One-shot trip (OSHT)
      settings: SourceProductName=Embedded Coder Support Package for Texas Instruments C2000 Processors  SourceProductBaseCode=TIC2000
  wires:
  "P-Regler mit Regelfehler Begrenzung Initial: k = 0.1, limiit = +/- 100 Sampletime 0.01"/1(pwm_out) -> "PWM Vorgabe für einen Motor "/1
  "P-Regler mit Regelfehler Begrenzung Initial: k = 0.1, limiit = +/- 100 Sampletime 0.01"/2(r/l_out) -> Drehrichtungsvorgabe für einen Motor/1
  Soll-Wert/1 -> "P-Regler mit Regelfehler Begrenzung Initial: k = 0.1, limiit = +/- 100 Sampletime 0.01"/2(y_soll)
  Ist-Wert/1 -> "P-Regler mit Regelfehler Begrenzung Initial: k = 0.1, limiit = +/- 100 Sampletime 0.01"/1(y_ist)

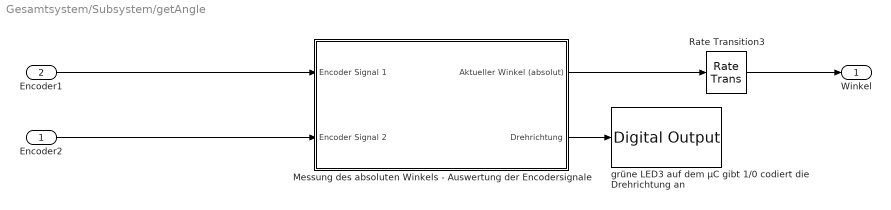
== system Gesamtsystem/Subsystem/getAngle ==
  Encoder2 : Inport
  Encoder1 : Inport  Port=2
  Messung des absoluten Winkels - Auswertung der Encodersignale : Subsystem
  Rate Transition3 : RateTransition  OutPortSampleTime=0.01
  grüne LED3 auf dem µC gibt 1/0 codiert die Drehrichtung an : c2833xlib/Digital Output  GPIO_Number=GPIO32~GPIO39  GPIO_Bit0=off  GPIO_BIT0_Toggle=off  GPIO_Bit1=off  GPIO_BIT1_Toggle=off  GPIO_Bit2=on  GPIO_BIT2_Toggle=off  GPIO_Bit3=off  GPIO_BIT3_Toggle=off  GPIO_Bit4=off  GPIO_BIT4_Toggle=off  GPIO_Bit5=off  GPIO_BIT5_Toggle=off  GPIO_Bit6=off  GPIO_BIT6_Toggle=off  GPIO_Bit7=off  GPIO_BIT7_Toggle=off
      settings: SourceProductName=Embedded Coder Support Package for Texas Instruments C2000 Processors  SourceProductBaseCode=TIC2000
  Winkel : Outport
  wires:
  Encoder1/1 -> Messung des absoluten Winkels - Auswertung der Encodersignale/1(Encoder Signal 1)
  Messung des absoluten Winkels - Auswertung der Encodersignale/2(Drehrichtung) -> grüne LED3 auf dem µC gibt 1/0 codiert die Drehrichtung an/1
  Messung des absoluten Winkels - Auswertung der Encodersignale/1(Aktueller Winkel (absolut)) -> Rate Transition3/1
  Encoder2/1 -> Messung des absoluten Winkels - Auswertung der Encodersignale/2(Encoder Signal 2)
  Rate Transition3/1 -> Winkel/1

== system Gesamtsystem/Nexonar-Positionsbestimmung/I2C Reset (behebt Stabilitätsprobleme der I2C-Verbindung)/I2C Reinitialisierung ==
  Trigger : TriggerPort  TriggerType=falling  VariantControl=(inherit)
  I2C Reinitialisierung : MATLAB Function  TreatAsAtomicUnit=on

== system Gesamtsystem/Nexonar-Positionsbestimmung/I2C Reset (behebt Stabilitätsprobleme der I2C-Verbindung)/I2C Reset ==
  Trigger : TriggerPort  VariantControl=(inherit)
  I2C Reset : MATLAB Function  TreatAsAtomicUnit=on

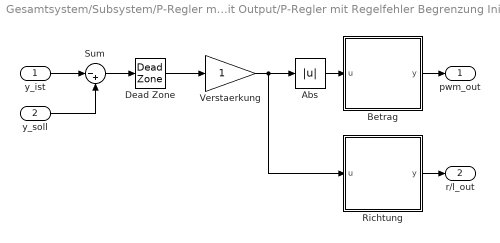
== system Gesamtsystem/Subsystem/P-Regler mit Output/P-Regler mit Regelfehler Begrenzung Initial: k = 0.1, limiit = +//- 100 Sampletime 0.01 ==
  y_ist : Inport
  y_soll : Inport  Port=2
  Abs : Abs  SampleTime=0.01
  Betrag : MATLAB Function  TreatAsAtomicUnit=on  SystemSampleTime=0.01
  Dead Zone : DeadZone  SampleTime=0.01  SaturateOnIntegerOverflow=on
  Richtung : MATLAB Function  TreatAsAtomicUnit=on  SystemSampleTime=0.01
  Sum : Sum  Inputs=|-+  SampleTime=0.01
  Verstaerkung : Gain  SampleTime=0.01
  pwm_out : Outport
  r/l_out : Outport  Port=2
  wires:
  Betrag/1(y) -> pwm_out/1
  Sum/1 -> Dead Zone/1
  Verstaerkung/1 -> Abs/1, Richtung/1(u)
  Dead Zone/1 -> Verstaerkung/1
  Abs/1 -> Betrag/1(u)
  y_soll/1 -> Sum/2
  Richtung/1(y) -> r/l_out/1
  y_ist/1 -> Sum/1

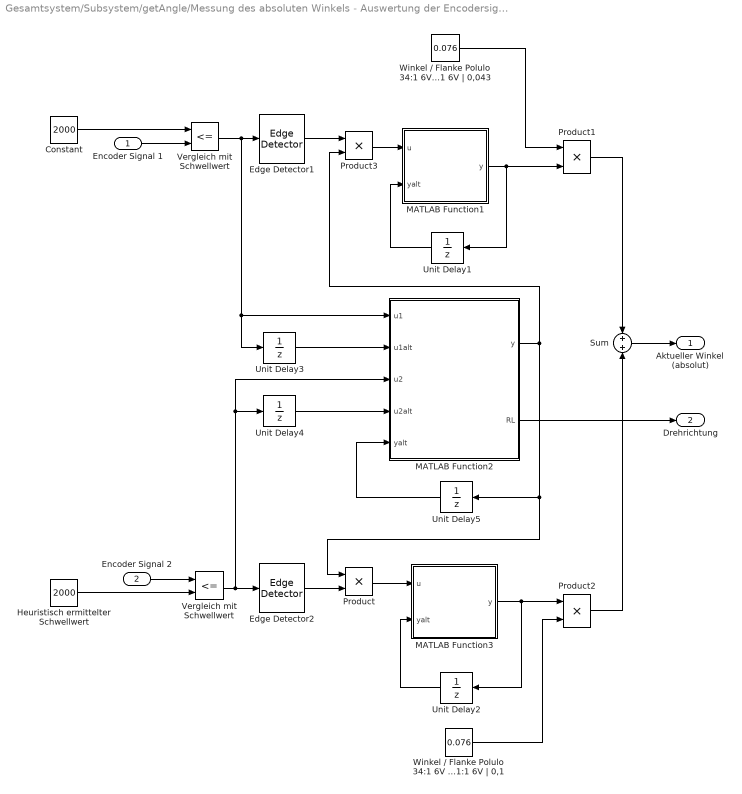
== system Gesamtsystem/Subsystem/getAngle/Messung des absoluten Winkels - Auswertung der Encodersignale ==
  Encoder Signal 1 : Inport
  Encoder Signal 2 : Inport  Port=2
  Constant : Constant  Value=2000
  Edge Detector1 : powerlib_extras/Control  Blocks/Edge Detector  model=Either  ic=0
  Edge Detector2 : powerlib_extras/Control  Blocks/Edge Detector  model=Either  ic=0
  Heuristisch ermittelter Schwellwert : Constant  Value=2000
  MATLAB Function1 : MATLAB Function  TreatAsAtomicUnit=on
  MATLAB Function2 : MATLAB Function  TreatAsAtomicUnit=on
  MATLAB Function3 : MATLAB Function  TreatAsAtomicUnit=on
  Product{,1..3} (4 alike) : Product  RndMeth=Zero
  Sum : Sum  Inputs=+|+
  Unit Delay{1..5} (5 alike) : UnitDelay  SampleTime=-1
  Vergleich mit Schwellwert : RelationalOperator  Operator=<=  OutDataTypeStr=boolean  RndMeth=Nearest
  Vergleich mit Schwellwert : RelationalOperator  Operator=<=  OutDataTypeStr=boolean  RndMeth=Nearest
  Winkel / Flanke Polulo 34:1 6V | 0,22 Polulo 74:1 6V | 0,1 Polulo 98:1 6V | 0,076 Polulo 171:1 6V | 0,043 : Constant  Value=0.076
  Winkel / Flanke Polulo 34:1 6V | 0,22 Polulo 74:1 6V | 0,1 Polulo 98:1 6V | 0,076 Polulo 171:1 6V | 0,1 : Constant  Value=0.076
  Aktueller Winkel (absolut) : Outport
  Drehrichtung : Outport  Port=2
  wires:
  Vergleich mit Schwellwert/1 -> Unit Delay4/1, MATLAB Function2/3(u2), Edge Detector2/1
  Sum/1 -> Aktueller Winkel (absolut)/1
  Vergleich mit Schwellwert/1 -> Edge Detector1/1, Unit Delay3/1, MATLAB Function2/1(u1)
  Heuristisch ermittelter Schwellwert/1 -> Vergleich mit Schwellwert/2
  Unit Delay2/1 -> MATLAB Function3/2(yalt)
  Encoder Signal 1/1 -> Vergleich mit Schwellwert/2
  MATLAB Function3/1(y) -> Unit Delay2/1, Product2/1
  Product1/1 -> Sum/1
  Constant/1 -> Vergleich mit Schwellwert/1
  Encoder Signal 2/1 -> Vergleich mit Schwellwert/1
  Product2/1 -> Sum/2
  Unit Delay1/1 -> MATLAB Function1/2(yalt)
  MATLAB Function1/1(y) -> Product1/2, Unit Delay1/1
  Winkel / Flanke Polulo 34:1 6V | 0,22 Polulo 74:1 6V | 0,1 Polulo 98:1 6V | 0,076 Polulo 171:1 6V | 0,043/1 -> Product1/1
  Product3/1 -> MATLAB Function1/1(u)
  Product/1 -> MATLAB Function3/1(u)
  Edge Detector1/1 -> Product3/1
  Unit Delay3/1 -> MATLAB Function2/2(u1alt)
  Unit Delay4/1 -> MATLAB Function2/4(u2alt)
  Edge Detector2/1 -> Product/2
  MATLAB Function2/1(y) -> Product/1, Unit Delay5/1, Product3/2
  Winkel / Flanke Polulo 34:1 6V | 0,22 Polulo 74:1 6V | 0,1 Polulo 98:1 6V | 0,076 Polulo 171:1 6V | 0,1/1 -> Product2/2
  MATLAB Function2/2(RL) -> Drehrichtung/1
  Unit Delay5/1 -> MATLAB Function2/5(yalt)

== stateflow chart Gesamtsystem/Nexonar-Positionsbestimmung/Chart1 ==
  state Daten_einlesen
  state x0
  state x1_1
    entry: int16z_bin[0] = int8z_1[0];
    int16z_bin[1] = int8z_1[1];
    int16z_bin[2] = int8z_1[2];
    int16z_bin[3] = int8z_1[3];
    int16z_bin[4] = int8z_1[4];
    int16z_bin[5] = int8z_1[5]
    int16z_bin[6] = int8z_1[6];
    int16z_bin[7] = int8z_1[7];
    int16z_bin[8] = int8z_2[0];
    int16z_bin[9] = int8z_2[1];
    int16z_bin[10] = int8z_2[2];
    int16z_bin[11] = int8z_2[3];
    int16z_bin[12] = int8z_2[4];
    int16z_bin[13] = int8z_2[5]
    int16z_bin[14] = int8z_2[6];
    int16z_bin[15] = int8z_2[7];
  x0 -> Daten_einlesen
  (default) -> x0
  Daten_einlesen -> x1_1
  x1_1 -> Daten_einlesen
  data: int8z_1 input size=8; int8z_2 input size=8; int16z_bin output size=16 =0

== matlab function Gesamtsystem/Navigationssystem [Einstellungen moeglich]/Positionsregelungssystem (Soll-Ist-Abgleich & PWM-Auswertung)/PWM-Vektorbetrag ==
  data: pwm_x input; pwm_out output; pwm_y input
function pwm_out = fcn(pwm_x, pwm_y)

pwm_out = round(sqrt(pwm_x * pwm_x + pwm_y * pwm_y));

== stateflow chart Gesamtsystem/Subsystem/Chart ==
  state init
    gateDirection = 0
    gatePWM = 50
  state wait
    gatePWM = 0
    gateDirection = 1
    movingCube = 0
  state close
    gateDirection = 0
  state open
    gatePWM = 50
    movingCube = 1
  (default) -> init
  init -> wait : [after(3,sec)]
  wait -> open : [signal == 1]
  open -> close : [after(0.3,sec)]
  close -> wait : [after(0.3, sec)]
  data: signal input; gatePWM output; gateDirection output; movingCube output single

== stateflow chart Gesamtsystem/Subsystem/Chart1 ==
  state firstEntry
    entry: angle = 300;
  note: StartWinkel, da Schieber nicht in Mitte stehen darf am Anfang. 5 Sekunden Zeit um das Bord einzuschalten
  state betterRightPosition
    angle = 220;
  state waitForCube
  state goToZero
    angle = 0;
    movingCube = 1
  state betterLeftPosition
    angle = -170;
  state closeGate
    signal = 0
  state wait
  state openGate
    signal = 1
    movingCube = 0
  state goToMagacin
    entry: angle = magacin;
  (default) -> firstEntry
  firstEntry -> waitForCube : [after(3,sec)]
  waitForCube -> betterRightPosition [order 1] : [(angle == 85)]
  betterRightPosition -> waitForCube
  waitForCube -> goToZero [order 3] : [magacin ~= -1]
  waitForCube -> betterLeftPosition [order 2] : [(angle == -40)]
  goToZero -> wait : [(inputAngle > -2) && (inputAngle < 2)]
  betterLeftPosition -> waitForCube
  closeGate -> waitForCube : [cubeFinished == 0]
  openGate -> closeGate : [after(0.5, sec)]
  wait -> goToMagacin : [after(0.4, sec)]
  goToMagacin -> openGate : [(inputAngle > (angle - 2)) && (inputAngle < (angle + 2))]
  data: inputAngle input; magacin input; angle output; signal output; movingCube output single; cubeFinished input
